simulink model "Braking_dynamics_model"  (R2024b)
settings: Solver=VariableStepAuto  StartTime=0.0  StopTime=6  FixedStep=0.01  RelTol=1e-3
values from neighbouring files (symbols this model uses):
  a = 1.8    [Longitudinal_braking_parameters.m]    (also in Longitudinal_driving_parameters.m)
  A = 1.25    [Longitudinal_braking_parameters.m]    (also in Longitudinal_driving_parameters.m)
  a1 = -1e-5    (= -1e-05)    [Longitudinal_braking_parameters.m]    (also in Longitudinal_driving_parameters.m)
  a2 = 1.25    [Longitudinal_braking_parameters.m]    (also in Longitudinal_driving_parameters.m)
  b = L-a    (= 1.7)    [Longitudinal_braking_parameters.m]    (also in Longitudinal_driving_parameters.m)
  B = 4.1576    [Longitudinal_braking_parameters.m]    (also in Longitudinal_driving_parameters.m = 5.7507)
  balance = 0.65    [Longitudinal_braking_parameters.m]
  C = 1.7180    (= 1.718)    [Longitudinal_braking_parameters.m]    (also in Longitudinal_driving_parameters.m = 1.2421)
  Cd = 0.6    [Longitudinal_braking_parameters.m]    (also in Longitudinal_driving_parameters.m = 0.4)
  Cz = 1.5    [Longitudinal_braking_parameters.m]
  g = 9.81    [Longitudinal_braking_parameters.m]    (also in Longitudinal_driving_parameters.m)
  h = 0.2    [Longitudinal_braking_parameters.m]    (also in Longitudinal_driving_parameters.m)
  Iwheel = 0.9    [Longitudinal_braking_parameters.m]    (also in Longitudinal_driving_parameters.m)
  L = 3.5    [Longitudinal_braking_parameters.m]    (also in Longitudinal_driving_parameters.m)
  m = 850    [Longitudinal_braking_parameters.m]    (also in Longitudinal_driving_parameters.m)
  r = 0.375    [Longitudinal_braking_parameters.m]    (also in Longitudinal_driving_parameters.m)
  rbrake = 3800    [Longitudinal_braking_parameters.m]
  rho = 1.225    [Longitudinal_braking_parameters.m]    (also in Longitudinal_driving_parameters.m)
settings Model: Creator=jayku  LastModifiedBy=jayku
settings DebuggingCC: AlgebraicLoopMsg=none

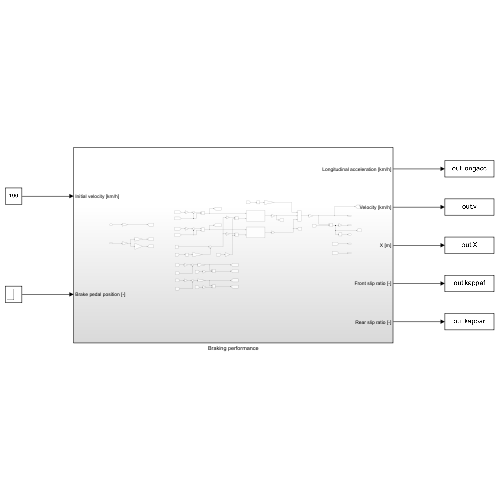
[thumbnail: Simulink's stored preview of the top-level diagram]
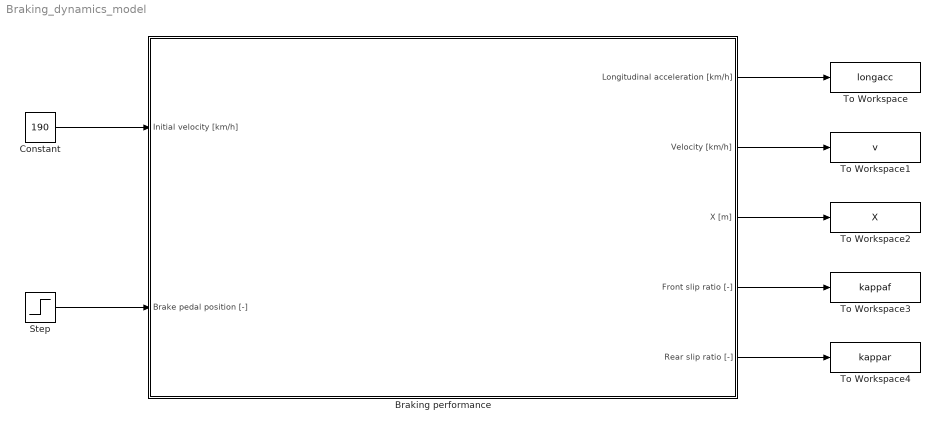
== system Braking_dynamics_model ==
  Braking performance : Subsystem
  Constant : Constant  Value=190
  Step : Step  Time=2.5  After=0.85  SampleTime=0
  To Workspace : ToWorkspace  VariableName=longacc  SaveFormat=Timeseries  SampleTime=-1
  To Workspace1 : ToWorkspace  VariableName=v  SaveFormat=Timeseries  SampleTime=-1
  To Workspace2 : ToWorkspace  VariableName=X  SaveFormat=Timeseries  SampleTime=-1
  To Workspace3 : ToWorkspace  VariableName=kappaf  SaveFormat=Timeseries  SampleTime=-1
  To Workspace4 : ToWorkspace  VariableName=kappar  SaveFormat=Timeseries  SampleTime=-1
  wires:
  Braking performance/1(Longitudinal acceleration [km/h]) -> To Workspace/1
  Braking performance/2(Velocity [km/h]) -> To Workspace1/1
  Braking performance/3(X [m]) -> To Workspace2/1
  Braking performance/4(Front slip ratio [-]) -> To Workspace3/1
  Braking performance/5(Rear slip ratio [-]) -> To Workspace4/1
  Constant/1 -> Braking performance/1(Initial velocity [km/h])
  Step/1 -> Braking performance/2(Brake pedal position [-])

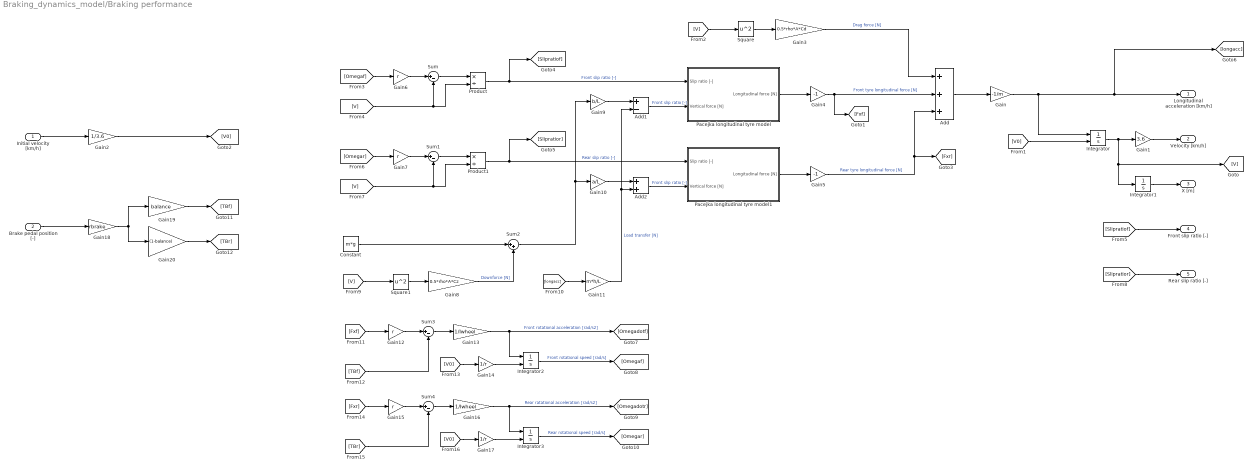
== system Braking_dynamics_model/Braking performance ==
  Initial velocity [km/h] : Inport
  Brake pedal position [-] : Inport  Port=2
  Add : Sum  Inputs=+++
  Add1 : Sum  Inputs=+-
  Add2 : Sum
  Constant : Constant  Value=m*g
  Gain : Gain  Gain=-1/m
  Gain1 : Gain  Gain=3.6
  Gain10 : Gain  Gain=a/L
  Gain11 : Gain  Gain=m*h/L
  Gain{6..7,12,15} (4 alike) : Gain  Gain=r
  Gain13 : Gain  Gain=1/Iwheel
  Gain14 : Gain  Gain=1/r
  Gain16 : Gain  Gain=1/Iwheel
  Gain17 : Gain  Gain=1/r
  Gain18 : Gain  Gain=rbrake
  Gain19 : Gain  Gain=balance
  Gain2 : Gain  Gain=1/3.6
  Gain20 : Gain  Gain=(1-balance)
  Gain3 : Gain  Gain=0.5*rho*A*Cd
  Gain4 : Gain  Gain=-1
  Gain5 : Gain  Gain=-1
  Gain8 : Gain  Gain=0.5*rho*A*Cz
  Gain9 : Gain  Gain=b/L
  Integrator : Integrator  InitialConditionSource=external
  Integrator1 : Integrator
  Integrator2 : Integrator  InitialConditionSource=external
  Integrator3 : Integrator  InitialConditionSource=external
  Pacejka longitudinal tyre model : Subsystem
  Pacejka longitudinal tyre model1 : Subsystem
  Product : Product  Inputs=*/
  Product1 : Product  Inputs=*/
  Square : Math  Operator=square
  Square1 : Math  Operator=square
  Sum{,1,3..4} (4 alike) : Sum  Inputs=|+-
  Sum2 : Sum  Inputs=|++
  Longitudinal acceleration [km/h] : Outport
  Velocity [km/h] : Outport  Port=2
  X [m] : Outport  Port=3
  Front slip ratio [-] : Outport  Port=4
  Rear slip ratio [-] : Outport  Port=5
  wires:
  Add/1 -> Gain/1
  Integrator/1 -> Integrator1/1, [V], Gain1/1
  Integrator1/1 -> X [m]/1
  Initial velocity [km/h]/1 -> Gain2/1
  Gain2/1 -> [V0]
  Gain1/1 -> Velocity [km/h]/1
  [V0] -> Integrator/2
  Gain3/1 -> Add/1  "Drag force [N]"
  Square/1 -> Gain3/1
  [V] -> Square/1
  Pacejka longitudinal tyre model/1(Longitudinal force [N]) -> Gain4/1
  Gain4/1 -> [Fxf], Add/2  "Front tyre longitudinal force [N]"
  Pacejka longitudinal tyre model1/1(Longitudinal force [N]) -> Gain5/1
  Gain5/1 -> [Fxr], Add/3  "Rear tyre longitudinal force [N]"
  [Omegaf] -> Gain6/1
  Gain6/1 -> Sum/1
  [V] -> Product/2, Sum/2
  Sum/1 -> Product/1
  Product/1 -> Pacejka longitudinal tyre model/1(Slip ratio [-]), [Slipratiof]  "Front slip ratio [-]"
  [Slipratiof] -> Front slip ratio [-]/1
  [V] -> Product1/2, Sum1/2
  Sum1/1 -> Product1/1
  Gain7/1 -> Sum1/1
  Product1/1 -> Pacejka longitudinal tyre model1/1(Slip ratio [-]), [Slipratior]  "Rear slip ratio [-]"
  [Omegar] -> Gain7/1
  [Slipratior] -> Rear slip ratio [-]/1
  Square1/1 -> Gain8/1
  [V] -> Square1/1
  Constant/1 -> Sum2/1
  Gain8/1 -> Sum2/2  "Downforce [N]"
  Gain9/1 -> Add1/1
  Gain10/1 -> Add2/1
  Sum2/1 -> Gain10/1, Gain9/1
  Add1/1 -> Pacejka longitudinal tyre model/2(Vertical force [N])  "Front slip ratio [-]"
  Add2/1 -> Pacejka longitudinal tyre model1/2(Vertical force [N])  "Front slip ratio [-]"
  Gain11/1 -> Add2/2, Add1/2  "Load transfer [N]"
  [longacc] -> Gain11/1
  [Fxf] -> Gain12/1
  Gain12/1 -> Sum3/1
  [TBf] -> Sum3/2
  Sum3/1 -> Gain13/1
  Gain13/1 -> Integrator2/1, [Omegadotf]  "Front rotational acceleration [rad/s2]"
  Integrator2/1 -> [Omegaf]  "Front rotational speed [rad/s]"
  Gain14/1 -> Integrator2/2
  [V0] -> Gain14/1
  Gain15/1 -> Sum4/1
  Sum4/1 -> Gain16/1
  Integrator3/1 -> [Omegar]  "Rear rotational speed [rad/s]"
  Gain16/1 -> Integrator3/1, [Omegadotr]  "Rear ratational acceleration [rad/s2]"
  [V0] -> Gain17/1
  Gain17/1 -> Integrator3/2
  [TBr] -> Sum4/2
  [Fxr] -> Gain15/1
  Brake pedal position [-]/1 -> Gain18/1
  Gain18/1 -> Gain20/1, Gain19/1
  Gain19/1 -> [TBf]
  Gain20/1 -> [TBr]
  Gain/1 -> Integrator/1, [longacc], Longitudinal acceleration [km/h]/1

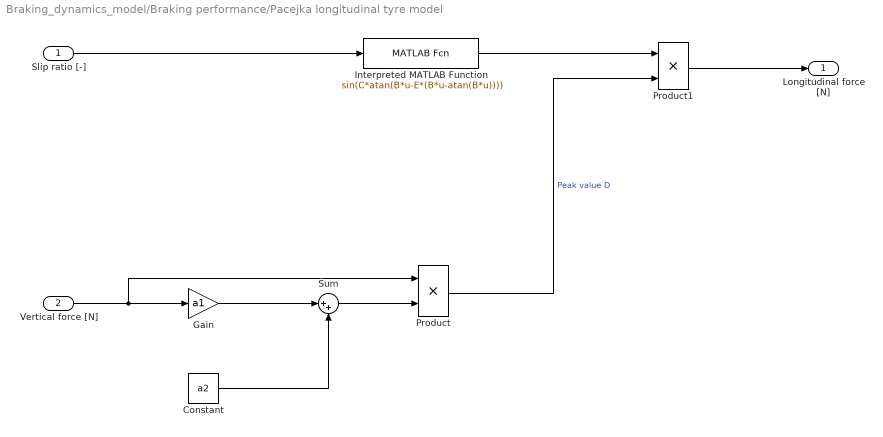
== system Braking_dynamics_model/Braking performance/Pacejka longitudinal tyre model ==
  Slip ratio [-] : Inport
  Vertical force [N] : Inport  Port=2
  Constant : Constant  Value=a2
  Gain : Gain  Gain=a1
  Interpreted MATLAB Function : MATLABFcn  MATLABFcn=sin(C*atan(B*u-E*(B*u-atan(B*u))))
  Product : Product
  Product1 : Product
  Sum : Sum  Inputs=|++
  Longitudinal force [N] : Outport
  wires:
  Slip ratio [-]/1 -> Interpreted MATLAB Function/1
  Vertical force [N]/1 -> Product/1, Gain/1
  Gain/1 -> Sum/1
  Constant/1 -> Sum/2
  Sum/1 -> Product/2
  Product/1 -> Product1/2  "Peak value D"
  Interpreted MATLAB Function/1 -> Product1/1
  Product1/1 -> Longitudinal force [N]/1

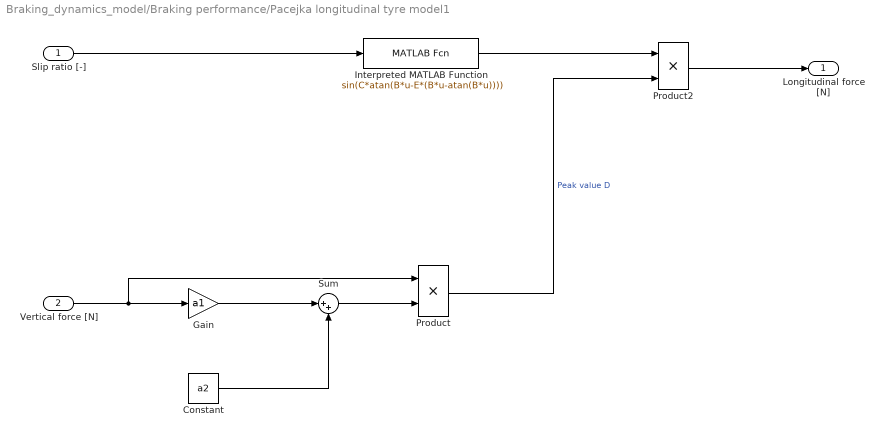
== system Braking_dynamics_model/Braking performance/Pacejka longitudinal tyre model1 ==
  Slip ratio [-] : Inport
  Vertical force [N] : Inport  Port=2
  Constant : Constant  Value=a2
  Gain : Gain  Gain=a1
  Interpreted MATLAB Function : MATLABFcn  MATLABFcn=sin(C*atan(B*u-E*(B*u-atan(B*u))))
  Product : Product
  Product2 : Product
  Sum : Sum  Inputs=|++
  Longitudinal force [N] : Outport
  wires:
  Slip ratio [-]/1 -> Interpreted MATLAB Function/1
  Vertical force [N]/1 -> Product/1, Gain/1
  Gain/1 -> Sum/1
  Constant/1 -> Sum/2
  Sum/1 -> Product/2
  Product/1 -> Product2/2  "Peak value D"
  Interpreted MATLAB Function/1 -> Product2/1
  Product2/1 -> Longitudinal force [N]/1
